simulink model "Q5Wheel1"  (R2021a)
settings: Solver=FixedStepAuto  StartTime=0.0  StopTime=130  FixedStep=0.001  RelTol=1e-3
values from neighbouring files (symbols this model uses):
  C = [cs1 0 0 -cs1 0 cs1*l1 0 ... (first row only)    [vibrtaion.m]
  K = [kt1+ks1 0 0 -ks1 0 ks1*l1 0 ... (first row only)    [vibrtaion.m]
  M = [m1 0   0  0  0  0  0 ... (first row only)    [vibrtaion.m]
settings Model: Creator=lenovo  LastModifiedBy=lenovo

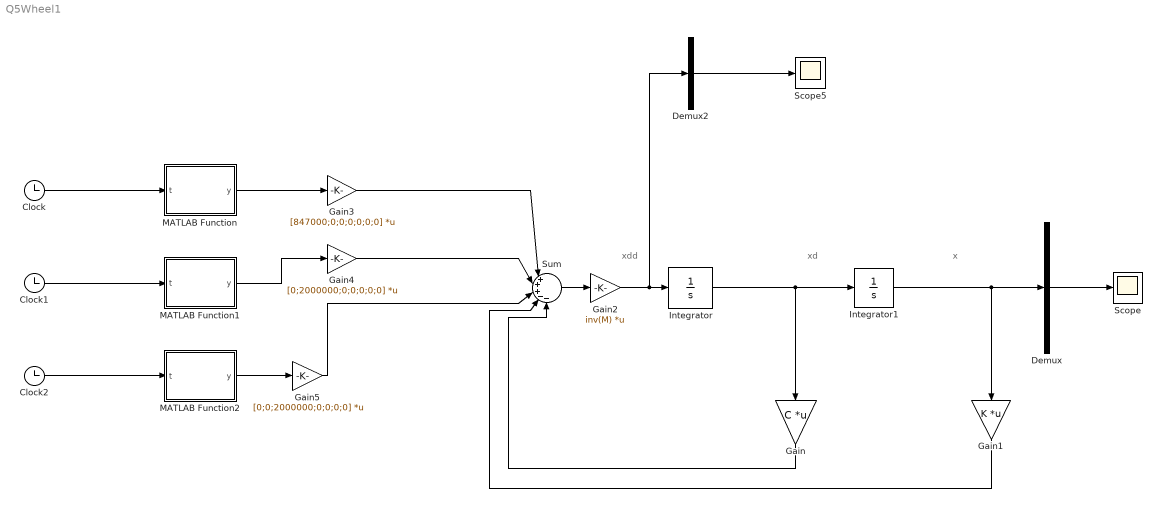
== system Q5Wheel1 ==
  note: x
  note: xdd
  note: xd
  Clock : Clock
  Clock1 : Clock
  Clock2 : Clock
  Demux : Demux  Outputs=7
  Demux2 : Demux  Outputs=7
  Gain : Gain  Gain=C  Multiplication=Matrix(K*u)
  Gain1 : Gain  Gain=K  Multiplication=Matrix(K*u)
  Gain2 : Gain  Gain=inv(M)  Multiplication=Matrix(K*u)
  Gain3 : Gain  Gain=[847000;0;0;0;0;0;0]  Multiplication=Matrix(K*u)
  Gain4 : Gain  Gain=[0;2000000;0;0;0;0;0]  Multiplication=Matrix(K*u)
  Gain5 : Gain  Gain=[0;0;2000000;0;0;0;0]  Multiplication=Matrix(K*u)
  Integrator : Integrator  InitialCondition=zeros(7,1)
  Integrator1 : Integrator  InitialCondition=zeros(7,1)
  MATLAB Function : MATLAB Function  TreatAsAtomicUnit=on
  MATLAB Function1 : MATLAB Function  TreatAsAtomicUnit=on
  MATLAB Function2 : MATLAB Function  TreatAsAtomicUnit=on
  Scope : Scope
  Scope5 : Scope
  Sum : Sum  Inputs=|+++--
  wires:
  Gain1/1 -> Sum/4
  Gain2/1 -> Demux2/1, Integrator/1
  Sum/1 -> Gain2/1
  Gain/1 -> Sum/5
  Demux/4 -> Scope/1
  Integrator/1 -> Gain/1, Integrator1/1
  Integrator1/1 -> Gain1/1, Demux/1
  Gain3/1 -> Sum/1
  MATLAB Function/1(y) -> Gain3/1
  Clock/1 -> MATLAB Function/1(t)
  Clock1/1 -> MATLAB Function1/1(t)
  MATLAB Function1/1(y) -> Gain4/1
  Gain4/1 -> Sum/2
  Clock2/1 -> MATLAB Function2/1(t)
  MATLAB Function2/1(y) -> Gain5/1
  Gain5/1 -> Sum/3
  Demux2/4 -> Scope5/1

== matlab function Q5Wheel1/MATLAB Function ==
  data: t input; y output
function y = Function(t)
if t>=0 && t<=0.30/v
y = 0.05*sin(((2*pi*v)/0.30)*t);
else y=0;
end

== matlab function Q5Wheel1/MATLAB Function2 ==
  data: t input; y output
function y = Function(t)
if t>=16.307/v && t<=(16.307/v)+(0.30/v)
y = 0.05*sin((2*pi*v)/0.3*(t-16.307/v));
else y=0;
end

== matlab function Q5Wheel1/MATLAB Function1 ==
  data: t input; y output
function y = Function(t)
if t>=(6/v) && t<=(6/v)+(0.30/v)
y = 0.05*sin((2*pi*v)/0.30*(t-6/v));
else y=0;
end
